simulink model "relop_test_tmp"  (Simulink 8.3)
settings: Solver=ode45  StartTime=0.0  StopTime=10.0  RelTol=1e-3
settings Model: Creator=arnaud  LastModifiedBy=hbourbou
settings OptimizationCC: ExpressionDepthLimit=2147483647
settings DebuggingCC: FcnCallInpInsideContextMsg=EnableAllAsWarning  FrameProcessingCompatibilityMsg=error

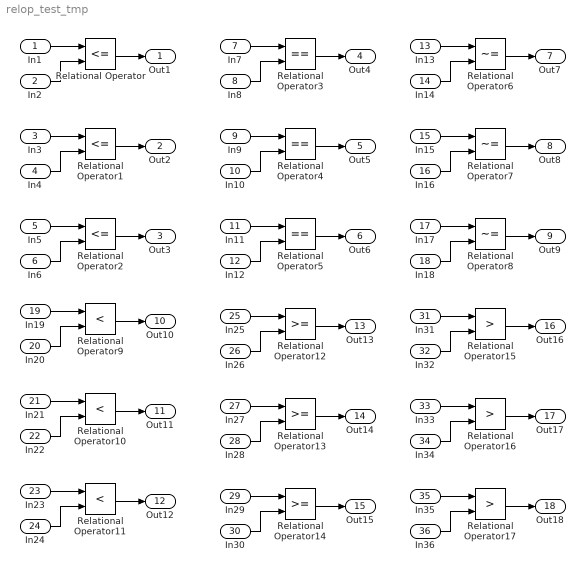
== system relop_test_tmp ==
  In1 : Inport  OutDataTypeStr=double  PortDimensions=1
  In2 : Inport  Port=2  OutDataTypeStr=double  PortDimensions=1
  In3 : Inport  Port=3  OutDataTypeStr=int8  PortDimensions=1
  In4 : Inport  Port=4  OutDataTypeStr=int8  PortDimensions=1
  In5 : Inport  Port=5  OutDataTypeStr=boolean  PortDimensions=1
  In6 : Inport  Port=6  OutDataTypeStr=single  PortDimensions=1
  In7 : Inport  Port=7  OutDataTypeStr=double  PortDimensions=1
  In8 : Inport  Port=8  OutDataTypeStr=double  PortDimensions=1
  In9 : Inport  Port=9  OutDataTypeStr=int8  PortDimensions=1
  In10 : Inport  Port=10  OutDataTypeStr=int8  PortDimensions=1
  In11 : Inport  Port=11  OutDataTypeStr=boolean
  In12 : Inport  Port=12  OutDataTypeStr=boolean
  In13 : Inport  Port=13  OutDataTypeStr=double
  In14 : Inport  Port=14  OutDataTypeStr=double
  In15 : Inport  Port=15  OutDataTypeStr=int8
  In16 : Inport  Port=16  OutDataTypeStr=int8
  In17 : Inport  Port=17  OutDataTypeStr=boolean
  In18 : Inport  Port=18  OutDataTypeStr=boolean
  In19 : Inport  Port=19  OutDataTypeStr=double
  In20 : Inport  Port=20  OutDataTypeStr=double
  In21 : Inport  Port=21  OutDataTypeStr=int8
  In22 : Inport  Port=22  OutDataTypeStr=int8
  In23 : Inport  Port=23  OutDataTypeStr=boolean
  In24 : Inport  Port=24  OutDataTypeStr=boolean
  In25 : Inport  Port=25  OutDataTypeStr=double
  In26 : Inport  Port=26  OutDataTypeStr=double
  In27 : Inport  Port=27  OutDataTypeStr=int8
  In28 : Inport  Port=28  OutDataTypeStr=int8
  In29 : Inport  Port=29  OutDataTypeStr=boolean
  In30 : Inport  Port=30  OutDataTypeStr=boolean
  In31 : Inport  Port=31  OutDataTypeStr=double
  In32 : Inport  Port=32  OutDataTypeStr=double
  In33 : Inport  Port=33  OutDataTypeStr=int8
  In34 : Inport  Port=34  OutDataTypeStr=int8
  In35 : Inport  Port=35  OutDataTypeStr=boolean
  In36 : Inport  Port=36  OutDataTypeStr=boolean
  Relational Operator : RelationalOperator  Operator=<=  OutDataTypeStr=boolean
  Relational Operator1 : RelationalOperator  Operator=<=  OutDataTypeStr=boolean
  Relational Operator10 : RelationalOperator  Operator=<  OutDataTypeStr=boolean
  Relational Operator11 : RelationalOperator  Operator=<  OutDataTypeStr=boolean
  Relational Operator12 : RelationalOperator  OutDataTypeStr=boolean
  Relational Operator13 : RelationalOperator  OutDataTypeStr=boolean
  Relational Operator14 : RelationalOperator  OutDataTypeStr=boolean
  Relational Operator15 : RelationalOperator  Operator=>  OutDataTypeStr=boolean
  Relational Operator16 : RelationalOperator  Operator=>  OutDataTypeStr=boolean
  Relational Operator17 : RelationalOperator  Operator=>  OutDataTypeStr=boolean
  Relational Operator2 : RelationalOperator  Operator=<=  OutDataTypeStr=boolean
  Relational Operator3 : RelationalOperator  Operator===  OutDataTypeStr=boolean
  Relational Operator4 : RelationalOperator  Operator===  OutDataTypeStr=boolean
  Relational Operator5 : RelationalOperator  Operator===  OutDataTypeStr=boolean
  Relational Operator6 : RelationalOperator  Operator=~=  OutDataTypeStr=boolean
  Relational Operator7 : RelationalOperator  Operator=~=  OutDataTypeStr=boolean
  Relational Operator8 : RelationalOperator  Operator=~=  OutDataTypeStr=boolean
  Relational Operator9 : RelationalOperator  Operator=<  OutDataTypeStr=boolean
  Out1 : Outport
  Out2 : Outport  Port=2
  Out3 : Outport  Port=3
  Out4 : Outport  Port=4
  Out5 : Outport  Port=5
  Out6 : Outport  Port=6
  Out7 : Outport  Port=7
  Out8 : Outport  Port=8
  Out9 : Outport  Port=9
  Out10 : Outport  Port=10
  Out11 : Outport  Port=11
  Out12 : Outport  Port=12
  Out13 : Outport  Port=13
  Out14 : Outport  Port=14
  Out15 : Outport  Port=15
  Out16 : Outport  Port=16
  Out17 : Outport  Port=17
  Out18 : Outport  Port=18
  wires:
  In1/1 -> Relational Operator/1
  Relational Operator/1 -> Out1/1
  In2/1 -> Relational Operator/2
  In3/1 -> Relational Operator1/1
  Relational Operator1/1 -> Out2/1
  In4/1 -> Relational Operator1/2
  In5/1 -> Relational Operator2/1
  Relational Operator2/1 -> Out3/1
  In6/1 -> Relational Operator2/2
  In7/1 -> Relational Operator3/1
  Relational Operator3/1 -> Out4/1
  In8/1 -> Relational Operator3/2
  In9/1 -> Relational Operator4/1
  Relational Operator4/1 -> Out5/1
  In10/1 -> Relational Operator4/2
  In11/1 -> Relational Operator5/1
  Relational Operator5/1 -> Out6/1
  In12/1 -> Relational Operator5/2
  In13/1 -> Relational Operator6/1
  Relational Operator6/1 -> Out7/1
  In14/1 -> Relational Operator6/2
  In15/1 -> Relational Operator7/1
  Relational Operator7/1 -> Out8/1
  In16/1 -> Relational Operator7/2
  In17/1 -> Relational Operator8/1
  Relational Operator8/1 -> Out9/1
  In18/1 -> Relational Operator8/2
  In19/1 -> Relational Operator9/1
  Relational Operator9/1 -> Out10/1
  In20/1 -> Relational Operator9/2
  In21/1 -> Relational Operator10/1
  Relational Operator10/1 -> Out11/1
  In22/1 -> Relational Operator10/2
  In23/1 -> Relational Operator11/1
  Relational Operator11/1 -> Out12/1
  In24/1 -> Relational Operator11/2
  In25/1 -> Relational Operator12/1
  Relational Operator12/1 -> Out13/1
  In26/1 -> Relational Operator12/2
  In27/1 -> Relational Operator13/1
  Relational Operator13/1 -> Out14/1
  In28/1 -> Relational Operator13/2
  In29/1 -> Relational Operator14/1
  Relational Operator14/1 -> Out15/1
  In30/1 -> Relational Operator14/2
  In31/1 -> Relational Operator15/1
  Relational Operator15/1 -> Out16/1
  In32/1 -> Relational Operator15/2
  In33/1 -> Relational Operator16/1
  Relational Operator16/1 -> Out17/1
  In34/1 -> Relational Operator16/2
  In35/1 -> Relational Operator17/1
  Relational Operator17/1 -> Out18/1
  In36/1 -> Relational Operator17/2
